simulink model "Transformation_V"  (R2020b)
settings: Solver=VariableStepAuto  StartTime=0.0  StopTime=10.0  RelTol=1e-3
values from neighbouring files (symbols this model uses):
  thetad = transpose(thetad)    [Transformation_VV.m]
  thetaV = transpose(thetaV)    [Transformation_VV.m]
settings Model: Creator=Jonathan van Zyl  LastModifiedBy=Jonathan van Zyl

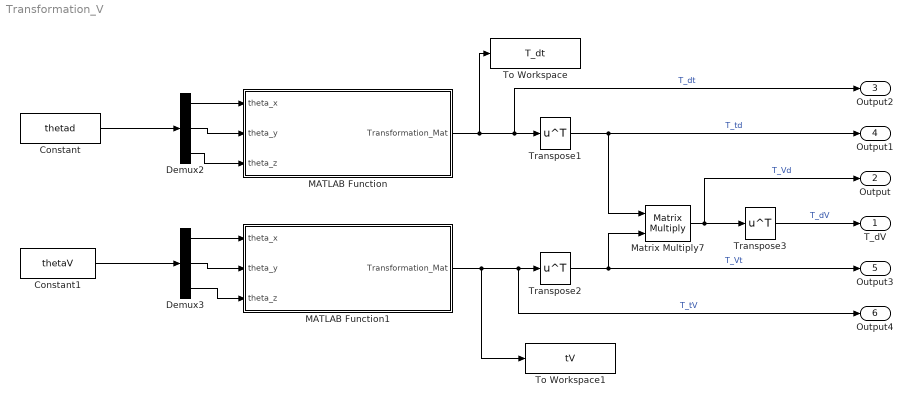
== system Transformation_V ==
  Constant : Constant  Value=thetad
  Constant1 : Constant  Value=thetaV
  Demux2 : Demux  Outputs=3
  Demux3 : Demux  Outputs=3
  MATLAB Function : MATLAB Function  TreatAsAtomicUnit=on
  MATLAB Function1 : MATLAB Function  TreatAsAtomicUnit=on
  Matrix Multiply7 : Product  Multiplication=Matrix(*)
  To Workspace : ToWorkspace  VariableName=T_dt  SampleTime=-1
      settings: MaxDataPoints=1
  To Workspace1 : ToWorkspace  VariableName=tV  SaveFormat=Timeseries  SampleTime=-1
  Transpose1 : Math  Operator=transpose  SaturateOnIntegerOverflow=on
  Transpose2 : Math  Operator=transpose  SaturateOnIntegerOverflow=on
  Transpose3 : Math  Operator=transpose  SaturateOnIntegerOverflow=on
  T_dV : Outport
  Output : Outport  Port=2
  Output2 : Outport  Port=3
  Output1 : Outport  Port=4
  Output3 : Outport  Port=5
  Output4 : Outport  Port=6
  wires:
  Constant/1 -> Demux2/1
  Demux3/1 -> MATLAB Function1/1(theta_x)
  Transpose3/1 -> T_dV/1  "T_dV"
  Demux3/2 -> MATLAB Function1/2(theta_y)
  Constant1/1 -> Demux3/1
  Demux3/3 -> MATLAB Function1/3(theta_z)
  Transpose2/1 -> Matrix Multiply7/2, Output3/1  "T_Vt"
  MATLAB Function1/1(Transformation_Mat) -> To Workspace1/1, Output4/1, Transpose2/1  "T_tV"
  Demux2/1 -> MATLAB Function/1(theta_x)
  Matrix Multiply7/1 -> Output/1, Transpose3/1  "T_Vd"
  Transpose1/1 -> Matrix Multiply7/1, Output1/1  "T_td"
  Demux2/3 -> MATLAB Function/3(theta_z)
  Demux2/2 -> MATLAB Function/2(theta_y)
  MATLAB Function/1(Transformation_Mat) -> To Workspace/1, Output2/1, Transpose1/1  "T_dt"

== matlab function Transformation_V/MATLAB Function1 ==
  data: theta_x input; Transformation_Mat output; theta_y input; theta_z input
function Transformation_Mat  = Euler(theta_x, theta_y, theta_z)

a = cos(theta_x)*cos(theta_z);
b = cos(theta_x)*sin(theta_z);
c = - sin(theta_x);
d = sin(theta_y)*sin(theta_x)*cos(theta_z) - cos(theta_y)*sin(theta_z);
e = sin(theta_y)*sin(theta_x)*sin(theta_z) + cos(theta_y)*cos(theta_z);
f = sin(theta_y)*cos(theta_x);
g = cos(theta_y)*sin(theta_x)*cos(theta_z) + sin(theta_y)*sin(theta_z);
h = cos(theta_y)*sin(theta_x)*sin(theta_z) - sin(theta_y)*cos(theta_z);
i = cos(theta_y)*cos(theta_x);

Transformation_Mat = [a b c;
    d e f;
    g h i];


end

== matlab function Transformation_V/MATLAB Function ==
  data: theta_x input; Transformation_Mat output; theta_y input; theta_z input
function Transformation_Mat  = Euler(theta_x, theta_y, theta_z)

a = cos(theta_x)*cos(theta_z);
b = cos(theta_x)*sin(theta_z);
c = - sin(theta_x);
d = sin(theta_y)*sin(theta_x)*cos(theta_z) - cos(theta_y)*sin(theta_z);
e = sin(theta_y)*sin(theta_x)*sin(theta_z) + cos(theta_y)*cos(theta_z);
f = sin(theta_y)*cos(theta_x);
g = cos(theta_y)*sin(theta_x)*cos(theta_z) + sin(theta_y)*sin(theta_z);
h = cos(theta_y)*sin(theta_x)*sin(theta_z) - sin(theta_y)*cos(theta_z);
i = cos(theta_y)*cos(theta_x);

Transformation_Mat = [a b c;
    d e f;
    g h i];


end
